simulink model "sixth"  (R2020b)
settings: Solver=FixedStepDiscrete  StartTime=0.0  StopTime=10.0  FixedStep=0.1  RelTol=1e-3
PostLoadFcn:
  | a0=2;
  | a1=-3;
  | a2=-4;
  | a3=5;
settings Model: Creator=priyaD  LastModifiedBy=priyaD

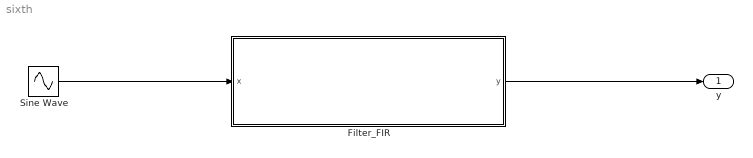
== system sixth ==
  Filter_FIR : Subsystem  TreatAsAtomicUnit=on
  Sine Wave : Sin  SampleTime=0
  y : Outport
  wires:
  Sine Wave/1 -> Filter_FIR/1(x)
  Filter_FIR/1(y) -> y/1

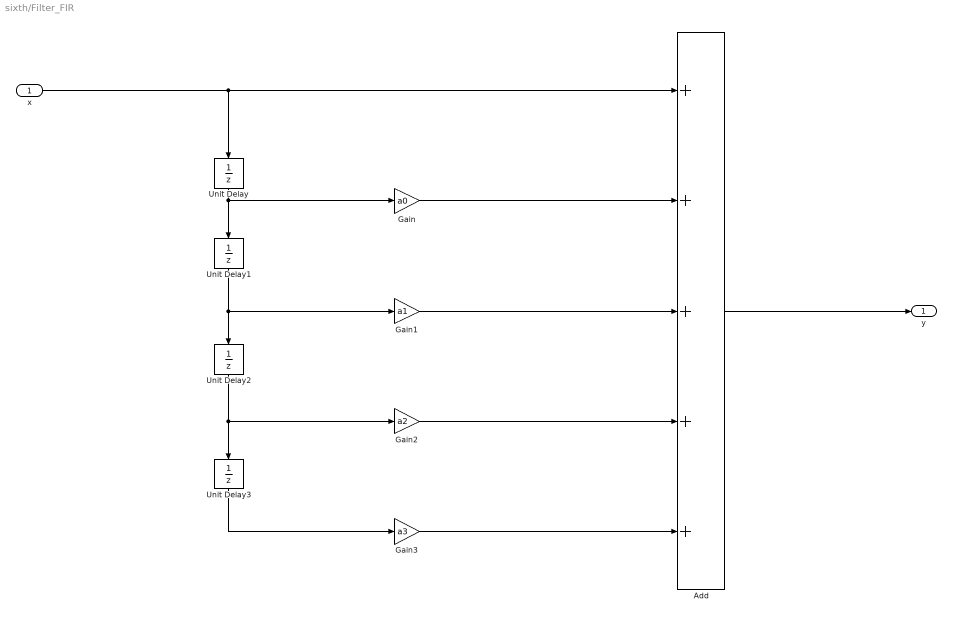
== system sixth/Filter_FIR ==
  x : Inport
  Add : Sum  Inputs=+++++
  Gain : Gain  Gain=a0
  Gain1 : Gain  Gain=a1
  Gain2 : Gain  Gain=a2
  Gain3 : Gain  Gain=a3
  Unit Delay{,1..3} (4 alike) : UnitDelay  SampleTime=-1  HasFrameUpgradeWarning=on
  y : Outport
  wires:
  Add/1 -> y/1
  Gain1/1 -> Add/3
  Unit Delay1/1 -> Gain1/1, Unit Delay2/1
  x/1 -> Unit Delay/1, Add/1
  Unit Delay3/1 -> Gain3/1
  Unit Delay2/1 -> Gain2/1, Unit Delay3/1
  Unit Delay/1 -> Gain/1, Unit Delay1/1
  Gain/1 -> Add/2
  Gain3/1 -> Add/5
  Gain2/1 -> Add/4
